simulink model "VCMGCM1962020b_v2"  (R2020b)
settings: Solver=FixedStepDiscrete  StartTime=0.0  StopTime=10.0  FixedStep=0.005  RelTol=1e-3  EnableMultiTasking=on
PreLoadFcn:
  | try, model_open; catch, disp('Error occurred while executing model pre-load callback: model_open.m'); disp('Please assure that the MATLAB working directory is set to the model directory before opening.'); end
InitFcn:
  | try, model_open; catch, end
undefined symbols (not defined in the file): Bridge, GCM, H, raptor_get_param_eval, raptor_get_safe_string, raptor_xcp_function
libraries: Blocks_lib x1165, Raptor_lib x665, simulink x62, VCM_lib x5
(part 11 of 23)

== system VCMGCM1962020b_v2/Fgnd/Sensors/CAN/Battery/DM01 ==
  note: The current .dbc, rev 6.0 has more messages than .dbc rev 4.0.
      | Have to figure out how these messages need to be routed.
  DiagEnbl : Inport
  Bus Creator : BusCreator  Inputs=2
  CANRxField5 : Blocks_lib/CANRxField  typ='uint8'  custom=off  custom_nam='---'  custom_units='---'
  CANRxMsgStatus : Blocks_lib/CANRxMsgStatus  samptime=samptime  custom=off  custom_nam='Name'  msgnam=DM01
  Ground : Ground
  Header : Blocks_lib/Header  width=Landscape  addtext=''
  raptor_can_rxmsg : Raptor_lib/CAN/raptor_can_rxmsg  canDefinition=struct('dbcFile', 'BMS dbc file_rev6.0.dbc','message', 'DM01','comment', '','signals', {{'Protect_Lamp','Amber_Warning_lamp','Red_Stop_Lamp','Malfunction_Indicator_Lamp','Flash_Protect_Lamp','Flash_Amber_Warning_Lamp','Flash_Red_Stop_Lamp','Flash_Malfunction_Indicator_Lamp','Suspect_Parameter_Number','Failure_Mode_Identifier','Occurence_Count','SPN_Conversion_Method'}},'enabled', [ 0 0 0 0 0 0 0 0 0 0 0 0;],'scaled', [ 1 1 1 1 1 1 1 1 1 1 1 1;],'canBus', 'bus','messageID', [ 419351283;],'idMask', [ 536870911;],'payloadMask', [],'payloadValue', [],'period', [ 0;],'mailbox', '''''','queueSize', [ 1;],'label', [ 1;],'ver', [ 2;],'showID', [ 0;],'showRaw', [ 0;],'fill', [ 0;],'editID', [ 0;],'signalOrder', [ 3;],'signalAscDes', [ 1;])  canBus=bus  mailbox=''  payloadMask=[]  payloadValue=[]  idMask=hex2dec('1FFFFFFF')  queueSize=1  showID=0  label=1  fill=0  id=419351283  showRaw=0  showAge=1  signalOrder=3  signalInfo={{struct('Name', 'Protect_Lamp','Startbit', [ 0;],'SignalSize', [ 4;],'ByteOrder', 'LittleEndian','ValueType', 'UNSIGNED','Class', 'uint8','Signed', [ 0;],'Factor', [ 1;],'Offset', [ 0;],'Min', [ 0;],'Max', [ 0;],'Units', '','Comment', '','StartBit', [ 0;]),struct('Name', 'Amber_Warning_lamp','Startbit', [ 0;],'SignalSize', [ 4;],'ByteOrder', 'LittleEndian','ValueType', 'UNSIGNED','Class', 'uint8','Signed', [ 0;],'Factor', [ 1;],'Offset', [ 0;],'Min', [ 0;],'Max', [ 0;],'Units', '','Comment', '','StartBit', [ 4;]),struct('Name', 'Red_Stop_Lamp','Startbit', [ 0;],'SignalSize', [ 4;],'ByteOrder', 'LittleEndian','ValueType', 'UNSIGNED','Class', 'uint8','Signed', [ 0;],'Factor', [ 1;],'Offset', [ 0;],'Min', [ 0;],'Max', [ 0;],'Units', '','Comment', '','StartBit', [ 8;]),struct('Name', 'Malfunction_Indicator_Lamp','Startbit', [ 0;],'SignalSize', [ 4;],'ByteOrder', 'LittleEndian','ValueType', 'UNSIGNED','Class', 'uint8','Signed', [ 0;],'Factor', [ 1;],'Offset', [ 0;],'Min', [ 0;],'Max', [ 0;],'Units', '','Comment', '','StartBit', [ 12;]),struct('Name', 'Flash_Protect_Lamp','Startbit', [ 0;],'SignalSize', [ 4;],'ByteOrder', 'LittleEndian','ValueType', 'UNSIGNED','Class', 'uint8','Signed', [ 0;],'Factor', [ 1;],'Offset', [ 0;],'Min', [ 0;],'Max', [ 0;],'Units', '','Comment', '','StartBit', [ 16;]),struct('Name', 'Flash_Amber_Warning_Lamp','Startbit', [ 0;],'SignalSize', [ 4;],'ByteOrder', 'LittleEndian','ValueType', 'UNSIGNED','Class', 'uint8','Signed', [ 0;],'Factor', [ 1;],'Offset', [ 0;],'Min', [ 0;],'Max', [ 0;],'Units', '','Comment', '','StartBit', [ 20;]),struct('Name', 'Flash_Red_Stop_Lamp','Startbit', [ 0;],'SignalSize', [ 4;],'ByteOrder', 'LittleEndian','ValueType', 'UNSIGNED','Class', 'uint8','Signed', [ 0;],'Factor', [ 1;],'Offset', [ 0;],'Min', [ 0;],'Max', [ 0;],'Units', '','Comment', '','StartBit', [ 24;]),struct('Name', 'Flash_Malfunction_Indicator_Lamp','Startbit', [ 0;],'SignalSize', [ 4;],'ByteOrder', 'LittleEndian','ValueType', 'UNSIGNED','Class', 'uint8','Signed', [ 0;],'Factor', [ 1;],'Offset', [ 0;],'Min', [ 0;],'Max', [ 0;],'Units', '','Comment', '','StartBit', [ 28;]),struct('Name', 'Suspect_Parameter_Number','Startbit', [ 0;],'SignalSize', [ 4;],'ByteOrder', 'LittleEndian','ValueType', 'UNSIGNED','Class', 'uint8','Signed', [ 0;],'Factor', [ 1;],'Offset', [ 0;],'Min', [ 0;],'Max', [ 0;],'Units', '','Comment', '','StartBit', [ 32;]),struct('Name', 'Failure_Mode_Identifier','Startbit', [ 0;],'SignalSize', [ 4;],'ByteOrder', 'LittleEndian','ValueType', 'UNSIGNED','Class', 'uint8','Signed', [ 0;],'Factor', [ 1;],'Offset', [ 0;],'Min', [ 0;],'Max', [ 0;],'Units', '','Comment', '','StartBit', [ 36;]),struct('Name', 'Occurence_Count','Startbit', [ 0;],'SignalSize', [ 4;],'ByteOrder', 'LittleEndian','ValueType', 'UNSIGNED','Class', 'uint8','Signed', [ 0;],'Factor', [ 1;],'Offset', [ 0;],'Min', [ 0;],'Max', [ 0;],'Units', '','Comment', '','StartBit', [ 40;]),struct('Name', 'SPN_Conversion_Method','Startbit', [ 0;],'SignalSize', [ 4;],'ByteOrder', 'LittleEndian','ValueType', 'UNSIGNED','Class', 'uint8','Signed', [ 0;],'Factor', [ 1;],'Offset', [ 0;],'Min', [ 0;],'Max', [ 0;],'Units', '','Comment', '','StartBit', [ 44;])}}
      settings: SourceProductName=Raptor
  Data : Outport  VectorParamsAs1DForOutWhenUnconnected=off
  wires:
  Bus Creator/1 -> Data/1  "MsgName"
  CANRxMsgStatus/1 -> Bus Creator/1
  DiagEnbl/1 -> CANRxMsgStatus/1
  raptor_can_rxmsg/1 -> CANRxMsgStatus/2  "Age"
  CANRxField5/1 -> Bus Creator/2
  Ground/1 -> CANRxField5/1  "Fault"

== system VCMGCM1962020b_v2/Fgnd/Sensors/CAN/Battery/HVES1_Data1 ==
  DiagEnbl : Inport
  Bus Creator : BusCreator  Inputs=5
  CANRxField{,1..3} (4 alike) : Blocks_lib/CANRxField  typ='double'  custom=off  custom_nam='---'  custom_units='---'
  CANRxMsgStatus : Blocks_lib/CANRxMsgStatus  samptime=samptime  custom=off  custom_nam='Name'  msgnam=HVES1_Data1
  Header : Blocks_lib/Header  width=Landscape  addtext=''
  raptor_can_rxmsg : Raptor_lib/CAN/raptor_can_rxmsg  canDefinition=struct('dbcFile', 'BMS dbc file_rev4.0.dbc','message', 'HVES1_Data1','comment', '20ms','signals', {{'Batt_Disch_Pow','Batt_Char_Pow','Batt_Voltage','Batt_Current'}},'enabled', [ 1 1 1 1;],'scaled', [ 1 1 1 1;],'canBus', 'bus','messageID', [ 217092339;],'idMask', [ 536870911;],'payloadMask', [],'payloadValue', [],'period', [ 0;],'mailbox', '''''','queueSize', [ 1;],'label', [ 1;],'ver', [ 2;],'showID', [ 0;],'showRaw', [ 0;],'showRawMsg', [ 0;],'showAge', [ 1;],'fill', [ 0;],'editID', [ 0;],'signalOrder', [ 3;],'signalAscDes', [ 1;])  canBus=bus  mailbox=''  payloadMask=[]  payloadValue=[]  idMask=hex2dec('1FFFFFFF')  queueSize=1  showID=0  label=1  fill=0  id=217092339  showRaw=0  showAge=1  signalOrder=3  signalInfo={{struct('Name', 'Batt_Disch_Pow','Startbit', [ 0;],'SignalSize', [ 16;],'ByteOrder', 'LittleEndian','ValueType', 'UNSIGNED','Class', 'uint16','Signed', [ 0;],'Factor', [ 0.05;],'Offset', [ 0;],'Min', [ 0;],'Max', [ 3212.75;],'Units', 'kW','Comment', '','StartBit', [ 0;]),struct('Name', 'Batt_Char_Pow','Startbit', [ 0;],'SignalSize', [ 16;],'ByteOrder', 'LittleEndian','ValueType', 'UNSIGNED','Class', 'uint16','Signed', [ 0;],'Factor', [ 0.05;],'Offset', [ 0;],'Min', [ 0;],'Max', [ 3212.75;],'Units', 'kW','Comment', '','StartBit', [ 16;]),struct('Name', 'Batt_Voltage','Startbit', [ 0;],'SignalSize', [ 16;],'ByteOrder', 'LittleEndian','ValueType', 'UNSIGNED','Class', 'uint16','Signed', [ 0;],'Factor', [ 0.05;],'Offset', [ 0;],'Min', [ 0;],'Max', [ 3212.75;],'Units', 'V','Comment', '','StartBit', [ 32;]),struct('Name', 'Batt_Current','Startbit', [ 0;],'SignalSize', [ 16;],'ByteOrder', 'LittleEndian','ValueType', 'UNSIGNED','Class', 'uint16','Signed', [ 0;],'Factor', [ 0.05;],'Offset', [ -1600;],'Min', [ -1600;],'Max', [ 1612.75;],'Units', 'A','Comment', '','StartBit', [ 48;])}}
      settings: SourceProductName=Raptor
  Data : Outport  VectorParamsAs1DForOutWhenUnconnected=off
  wires:
  Bus Creator/1 -> Data/1  "MsgName"
  raptor_can_rxmsg/2 -> CANRxField/1  "Batt_Disch_Pow"
  CANRxMsgStatus/1 -> Bus Creator/1
  CANRxField/1 -> Bus Creator/2
  DiagEnbl/1 -> CANRxMsgStatus/1
  raptor_can_rxmsg/1 -> CANRxMsgStatus/2  "Age"
  raptor_can_rxmsg/5 -> CANRxField3/1  "Batt_Current"
  raptor_can_rxmsg/3 -> CANRxField1/1  "Batt_Char_Pow"
  raptor_can_rxmsg/4 -> CANRxField2/1  "Batt_Voltage"
  CANRxField1/1 -> Bus Creator/3
  CANRxField2/1 -> Bus Creator/4
  CANRxField3/1 -> Bus Creator/5

== system VCMGCM1962020b_v2/Fgnd/Sensors/CAN/Battery/HVES1_Data10 ==
  DiagEnbl : Inport
  Bus Creator : BusCreator  Inputs=2
  CANRxField : Blocks_lib/CANRxField  typ='double'  custom=off  custom_nam='---'  custom_units='---'
  CANRxMsgStatus : Blocks_lib/CANRxMsgStatus  samptime=samptime  custom=off  custom_nam='Name'  msgnam=HVES1_Data10
  Header : Blocks_lib/Header  width=Landscape  addtext=''
  raptor_can_rxmsg : Raptor_lib/CAN/raptor_can_rxmsg  canDefinition=struct('dbcFile', 'BMS dbc file_rev4.0.dbc','message', 'HVES1_Data10','comment', '100ms','signals', {{'PSV_ISO_Measurement'}},'enabled', [ 1;],'scaled', [ 1;],'canBus', 'bus','messageID', [ 217124083;],'idMask', [ 536870911;],'payloadMask', [],'payloadValue', [],'period', [ 0;],'mailbox', '''''','queueSize', [ 1;],'label', [ 1;],'ver', [ 2;],'showID', [ 0;],'showRaw', [ 0;],'showRawMsg', [ 0;],'showAge', [ 1;],'fill', [ 0;],'editID', [ 0;],'signalOrder', [ 3;],'signalAscDes', [ 1;])  canBus=bus  mailbox=''  payloadMask=[]  payloadValue=[]  idMask=hex2dec('1FFFFFFF')  queueSize=1  showID=0  label=1  fill=0  id=217124083  showRaw=0  showAge=1  signalOrder=3  signalInfo={{struct('Name', 'PSV_ISO_Measurement','Startbit', [ 0;],'SignalSize', [ 16;],'ByteOrder', 'LittleEndian','ValueType', 'UNSIGNED','Class', 'uint16','Signed', [ 0;],'Factor', [ 0.1;],'Offset', [ 0;],'Min', [ 0;],'Max', [ 6425.5;],'Units', 'ohm/volt','Comment', '','StartBit', [ 48;])}}
      settings: SourceProductName=Raptor
  Data : Outport  VectorParamsAs1DForOutWhenUnconnected=off
  wires:
  Bus Creator/1 -> Data/1  "MsgName"
  raptor_can_rxmsg/2 -> CANRxField/1  "PSV_ISO_Measurement"
  CANRxMsgStatus/1 -> Bus Creator/1
  CANRxField/1 -> Bus Creator/2
  DiagEnbl/1 -> CANRxMsgStatus/1
  raptor_can_rxmsg/1 -> CANRxMsgStatus/2  "Age"

== system VCMGCM1962020b_v2/Fgnd/Sensors/CAN/Battery/HVES1_Data2 ==
  DiagEnbl : Inport
  Bus Creator : BusCreator  Inputs=4
  CANRxField : Blocks_lib/CANRxField  typ='double'  custom=off  custom_nam='---'  custom_units='---'
  CANRxField1 : Blocks_lib/CANRxField  typ='double'  custom=off  custom_nam='---'  custom_units='---'
  CANRxField2 : Blocks_lib/CANRxField  typ='double'  custom=off  custom_nam='---'  custom_units='---'
  CANRxMsgStatus : Blocks_lib/CANRxMsgStatus  samptime=samptime  custom=off  custom_nam='Name'  msgnam=HVES1_Data2
  Header : Blocks_lib/Header  width=Landscape  addtext=''
  raptor_can_rxmsg : Raptor_lib/CAN/raptor_can_rxmsg  canDefinition=struct('dbcFile', 'BMS dbc file_rev4.0.dbc','message', 'HVES1_Data2','comment', '20ms','signals', {{'Batt_SOC','Batt_Cell_Volt_High','Batt_Cell_Volt_Low'}},'enabled', [ 1 1 1;],'scaled', [ 1 1 1;],'canBus', 'bus','messageID', [ 217092595;],'idMask', [ 536870911;],'payloadMask', [],'payloadValue', [],'period', [ 0;],'mailbox', '''''','queueSize', [ 1;],'label', [ 1;],'ver', [ 2;],'showID', [ 0;],'showRaw', [ 0;],'showRawMsg', [ 0;],'showAge', [ 1;],'fill', [ 0;],'editID', [ 0;],'signalOrder', [ 3;],'signalAscDes', [ 1;])  canBus=bus  mailbox=''  payloadMask=[]  payloadValue=[]  idMask=hex2dec('1FFFFFFF')  queueSize=1  showID=0  label=1  fill=0  id=217092595  showRaw=0  showAge=1  signalOrder=3  signalInfo={{struct('Name', 'Batt_SOC','Startbit', [ 0;],'SignalSize', [ 16;],'ByteOrder', 'LittleEndian','ValueType', 'UNSIGNED','Class', 'uint16','Signed', [ 0;],'Factor', [ 0.0015625;],'Offset', [ 0;],'Min', [ 0;],'Max', [ 100.3984;],'Units', '%','Comment', '','StartBit', [ 0;]),struct('Name', 'Batt_Cell_Volt_High','Startbit', [ 0;],'SignalSize', [ 16;],'ByteOrder', 'LittleEndian','ValueType', 'UNSIGNED','Class', 'uint16','Signed', [ 0;],'Factor', [ 0.001;],'Offset', [ 0;],'Min', [ 0;],'Max', [ 64.225;],'Units', 'V','Comment', '','StartBit', [ 16;]),struct('Name', 'Batt_Cell_Volt_Low','Startbit', [ 0;],'SignalSize', [ 16;],'ByteOrder', 'LittleEndian','ValueType', 'UNSIGNED','Class', 'uint16','Signed', [ 0;],'Factor', [ 0.001;],'Offset', [ 0;],'Min', [ 0;],'Max', [ 64.225;],'Units', 'V','Comment', '','StartBit', [ 32;])}}
      settings: SourceProductName=Raptor
  Data : Outport  VectorParamsAs1DForOutWhenUnconnected=off
  wires:
  Bus Creator/1 -> Data/1  "MsgName"
  raptor_can_rxmsg/2 -> CANRxField/1  "Batt_SOC"
  CANRxMsgStatus/1 -> Bus Creator/1
  CANRxField/1 -> Bus Creator/2
  DiagEnbl/1 -> CANRxMsgStatus/1
  raptor_can_rxmsg/1 -> CANRxMsgStatus/2  "Age"
  raptor_can_rxmsg/3 -> CANRxField1/1  "Batt_Cell_Volt_High"
  raptor_can_rxmsg/4 -> CANRxField2/1  "Batt_Cell_Volt_Low"
  CANRxField1/1 -> Bus Creator/3
  CANRxField2/1 -> Bus Creator/4

== system VCMGCM1962020b_v2/Fgnd/Sensors/CAN/Battery/HVES1_Data3 ==
  DiagEnbl : Inport
  Bus Creator : BusCreator  Inputs=4
  CANRxField : Blocks_lib/CANRxField  typ='double'  custom=off  custom_nam='---'  custom_units='---'
  CANRxField1 : Blocks_lib/CANRxField  typ='double'  custom=off  custom_nam='---'  custom_units='---'
  CANRxField2 : Blocks_lib/CANRxField  typ='double'  custom=off  custom_nam='---'  custom_units='---'
  CANRxMsgStatus : Blocks_lib/CANRxMsgStatus  samptime=samptime  custom=off  custom_nam='Name'  msgnam=HVES1_Data3
  Header : Blocks_lib/Header  width=Landscape  addtext=''
  raptor_can_rxmsg : Raptor_lib/CAN/raptor_can_rxmsg  canDefinition=struct('dbcFile', 'BMS dbc file_rev4.0.dbc','message', 'HVES1_Data3','comment', '20ms','signals', {{'Batt_Max_Cell_Temp','Batt_Min_Cell_Temp','Batt_Ave_Cell_Temp'}},'enabled', [ 1 1 1;],'scaled', [ 1 1 1;],'canBus', 'bus','messageID', [ 217092851;],'idMask', [ 536870911;],'payloadMask', [],'payloadValue', [],'period', [ 0;],'mailbox', '''''','queueSize', [ 1;],'label', [ 1;],'ver', [ 2;],'showID', [ 0;],'showRaw', [ 0;],'showRawMsg', [ 0;],'showAge', [ 1;],'fill', [ 0;],'editID', [ 0;],'signalOrder', [ 3;],'signalAscDes', [ 1;])  canBus=bus  mailbox=''  payloadMask=[]  payloadValue=[]  idMask=hex2dec('1FFFFFFF')  queueSize=1  showID=0  label=1  fill=0  id=217092851  showRaw=0  showAge=1  signalOrder=3  signalInfo={{struct('Name', 'Batt_Max_Cell_Temp','Startbit', [ 0;],'SignalSize', [ 16;],'ByteOrder', 'LittleEndian','ValueType', 'UNSIGNED','Class', 'uint16','Signed', [ 0;],'Factor', [ 0.03125;],'Offset', [ -273;],'Min', [ -273;],'Max', [ 1734.9687;],'Units', 'C','Comment', '','StartBit', [ 0;]),struct('Name', 'Batt_Min_Cell_Temp','Startbit', [ 0;],'SignalSize', [ 16;],'ByteOrder', 'LittleEndian','ValueType', 'UNSIGNED','Class', 'uint16','Signed', [ 0;],'Factor', [ 0.03125;],'Offset', [ -273;],'Min', [ -273;],'Max', [ 1734.9688;],'Units', 'C','Comment', '','StartBit', [ 16;]),struct('Name', 'Batt_Ave_Cell_Temp','Startbit', [ 0;],'SignalSize', [ 16;],'ByteOrder', 'LittleEndian','ValueType', 'UNSIGNED','Class', 'uint16','Signed', [ 0;],'Factor', [ 0.03125;],'Offset', [ -273;],'Min', [ -273;],'Max', [ 1734.9688;],'Units', 'C','Comment', '','StartBit', [ 32;])}}
      settings: SourceProductName=Raptor
  Data : Outport  VectorParamsAs1DForOutWhenUnconnected=off
  wires:
  Bus Creator/1 -> Data/1  "MsgName"
  raptor_can_rxmsg/2 -> CANRxField/1  "Batt_Max_Cell_Temp"
  CANRxMsgStatus/1 -> Bus Creator/1
  CANRxField/1 -> Bus Creator/2
  DiagEnbl/1 -> CANRxMsgStatus/1
  raptor_can_rxmsg/1 -> CANRxMsgStatus/2  "Age"
  raptor_can_rxmsg/3 -> CANRxField1/1  "Batt_Min_Cell_Temp"
  raptor_can_rxmsg/4 -> CANRxField2/1  "Batt_Ave_Cell_Temp"
  CANRxField1/1 -> Bus Creator/3
  CANRxField2/1 -> Bus Creator/4

== system VCMGCM1962020b_v2/Fgnd/Sensors/CAN/Battery/HVES1_Data4 ==
  DiagEnbl : Inport
  Bus Creator : BusCreator  Inputs=3
  CANRxField : Blocks_lib/CANRxField  typ='double'  custom=off  custom_nam='---'  custom_units='---'
  CANRxField1 : Blocks_lib/CANRxField  typ='double'  custom=off  custom_nam='---'  custom_units='---'
  CANRxMsgStatus : Blocks_lib/CANRxMsgStatus  samptime=samptime  custom=off  custom_nam='Name'  msgnam=HVES1_Data4
  Header : Blocks_lib/Header  width=Landscape  addtext=''
  raptor_can_rxmsg : Raptor_lib/CAN/raptor_can_rxmsg  canDefinition=struct('dbcFile', 'BMS dbc file_rev4.0.dbc','message', 'HVES1_Data4','comment', '100ms','signals', {{'Batt_Disch_cap','Batt_Charge_cap'}},'enabled', [ 1 1;],'scaled', [ 1 1;],'canBus', 'bus','messageID', [ 217093107;],'idMask', [ 536870911;],'payloadMask', [],'payloadValue', [],'period', [ 0;],'mailbox', '''''','queueSize', [ 1;],'label', [ 1;],'ver', [ 2;],'showID', [ 0;],'showRaw', [ 0;],'showRawMsg', [ 0;],'showAge', [ 1;],'fill', [ 0;],'editID', [ 0;],'signalOrder', [ 3;],'signalAscDes', [ 1;])  canBus=bus  mailbox=''  payloadMask=[]  payloadValue=[]  idMask=hex2dec('1FFFFFFF')  queueSize=1  showID=0  label=1  fill=0  id=217093107  showRaw=0  showAge=1  signalOrder=3  signalInfo={{struct('Name', 'Batt_Disch_cap','Startbit', [ 0;],'SignalSize', [ 16;],'ByteOrder', 'LittleEndian','ValueType', 'UNSIGNED','Class', 'uint16','Signed', [ 0;],'Factor', [ 0.01;],'Offset', [ 0;],'Min', [ 0;],'Max', [ 642.55;],'Units', 'Ah','Comment', '','StartBit', [ 0;]),struct('Name', 'Batt_Charge_cap','Startbit', [ 0;],'SignalSize', [ 16;],'ByteOrder', 'LittleEndian','ValueType', 'UNSIGNED','Class', 'uint16','Signed', [ 0;],'Factor', [ 0.01;],'Offset', [ 0;],'Min', [ 0;],'Max', [ 642.55;],'Units', 'Ah','Comment', '','StartBit', [ 16;])}}
      settings: SourceProductName=Raptor
  Data : Outport  VectorParamsAs1DForOutWhenUnconnected=off
  wires:
  Bus Creator/1 -> Data/1  "MsgName"
  raptor_can_rxmsg/2 -> CANRxField/1  "Batt_Disch_cap"
  CANRxMsgStatus/1 -> Bus Creator/1
  CANRxField/1 -> Bus Creator/2
  DiagEnbl/1 -> CANRxMsgStatus/1
  raptor_can_rxmsg/1 -> CANRxMsgStatus/2  "Age"
  raptor_can_rxmsg/3 -> CANRxField1/1  "Batt_Charge_cap"
  CANRxField1/1 -> Bus Creator/3

== system VCMGCM1962020b_v2/Fgnd/Sensors/CAN/Battery/HVES1_Data5 ==
  DiagEnbl : Inport
  Bus Creator : BusCreator  Inputs=3
  CANRxField : Blocks_lib/CANRxField  typ='double'  custom=off  custom_nam='---'  custom_units='---'
  CANRxField1 : Blocks_lib/CANRxField  typ='double'  custom=off  custom_nam='---'  custom_units='---'
  CANRxMsgStatus : Blocks_lib/CANRxMsgStatus  samptime=samptime  custom=off  custom_nam='Name'  msgnam=HVES1_Data5
  Header : Blocks_lib/Header  width=Landscape  addtext=''
  raptor_can_rxmsg : Raptor_lib/CAN/raptor_can_rxmsg  canDefinition=struct('dbcFile', 'BMS dbc file_rev4.0.dbc','message', 'HVES1_Data5','comment', '20ms','signals', {{'Batt_Disch_Curr_Lim','Batt_Charge_Curr_Lim'}},'enabled', [ 1 1;],'scaled', [ 1 1;],'canBus', 'bus','messageID', [ 217093363;],'idMask', [ 536870911;],'payloadMask', [],'payloadValue', [],'period', [ 0;],'mailbox', '''''','queueSize', [ 1;],'label', [ 1;],'ver', [ 2;],'showID', [ 0;],'showRaw', [ 0;],'showRawMsg', [ 0;],'showAge', [ 1;],'fill', [ 0;],'editID', [ 0;],'signalOrder', [ 3;],'signalAscDes', [ 1;])  canBus=bus  mailbox=''  payloadMask=[]  payloadValue=[]  idMask=hex2dec('1FFFFFFF')  queueSize=1  showID=0  label=1  fill=0  id=217093363  showRaw=0  showAge=1  signalOrder=3  signalInfo={{struct('Name', 'Batt_Disch_Curr_Lim','Startbit', [ 0;],'SignalSize', [ 16;],'ByteOrder', 'LittleEndian','ValueType', 'UNSIGNED','Class', 'uint16','Signed', [ 0;],'Factor', [ 0.05;],'Offset', [ -1600;],'Min', [ -1600;],'Max', [ 1612.75;],'Units', 'A','Comment', '','StartBit', [ 0;]),struct('Name', 'Batt_Charge_Curr_Lim','Startbit', [ 0;],'SignalSize', [ 16;],'ByteOrder', 'LittleEndian','ValueType', 'UNSIGNED','Class', 'uint16','Signed', [ 0;],'Factor', [ 0.05;],'Offset', [ -1600;],'Min', [ -1600;],'Max', [ 1612.75;],'Units', 'A','Comment', '','StartBit', [ 16;])}}
      settings: SourceProductName=Raptor
  Data : Outport  VectorParamsAs1DForOutWhenUnconnected=off
  wires:
  Bus Creator/1 -> Data/1  "MsgName"
  raptor_can_rxmsg/2 -> CANRxField/1  "Batt_Disch_Curr_Lim"
  CANRxMsgStatus/1 -> Bus Creator/1
  CANRxField/1 -> Bus Creator/2
  DiagEnbl/1 -> CANRxMsgStatus/1
  raptor_can_rxmsg/1 -> CANRxMsgStatus/2  "Age"
  raptor_can_rxmsg/3 -> CANRxField1/1  "Batt_Charge_Curr_Lim"
  CANRxField1/1 -> Bus Creator/3

== system VCMGCM1962020b_v2/Fgnd/Sensors/CAN/Battery/HVES1_Data6 ==
  DiagEnbl : Inport
  Bus Creator : BusCreator  Inputs=4
  CANRxField : Blocks_lib/CANRxField  typ='double'  custom=off  custom_nam='---'  custom_units='---'
  CANRxField1 : Blocks_lib/CANRxField  typ='double'  custom=off  custom_nam='---'  custom_units='---'
  CANRxField2 : Blocks_lib/CANRxField  typ='double'  custom=off  custom_nam='---'  custom_units='---'
  CANRxMsgStatus : Blocks_lib/CANRxMsgStatus  samptime=samptime  custom=off  custom_nam='Name'  msgnam=HVES1_Data6
  Header : Blocks_lib/Header  width=Landscape  addtext=''
  raptor_can_rxmsg : Raptor_lib/CAN/raptor_can_rxmsg  canDefinition=struct('dbcFile', 'BMS dbc file_rev4.0.dbc','message', 'HVES1_Data6','comment', '100ms','signals', {{'Batt_Bus_Vol','Batt_inlet_cool_temp','Batt_outlet_cool_temp'}},'enabled', [ 1 1 1;],'scaled', [ 1 1 1;],'canBus', 'bus','messageID', [ 217093619;],'idMask', [ 536870911;],'payloadMask', [],'payloadValue', [],'period', [ 0;],'mailbox', '''''','queueSize', [ 1;],'label', [ 1;],'ver', [ 2;],'showID', [ 0;],'showRaw', [ 0;],'showRawMsg', [ 0;],'showAge', [ 1;],'fill', [ 0;],'editID', [ 0;],'signalOrder', [ 3;],'signalAscDes', [ 1;])  canBus=bus  mailbox=''  payloadMask=[]  payloadValue=[]  idMask=hex2dec('1FFFFFFF')  queueSize=1  showID=0  label=1  fill=0  id=217093619  showRaw=0  showAge=1  signalOrder=3  signalInfo={{struct('Name', 'Batt_Bus_Vol','Startbit', [ 0;],'SignalSize', [ 16;],'ByteOrder', 'LittleEndian','ValueType', 'UNSIGNED','Class', 'uint16','Signed', [ 0;],'Factor', [ 0.05;],'Offset', [ 0;],'Min', [ 0;],'Max', [ 3212.75;],'Units', 'V','Comment', '','StartBit', [ 0;]),struct('Name', 'Batt_inlet_cool_temp','Startbit', [ 0;],'SignalSize', [ 8;],'ByteOrder', 'LittleEndian','ValueType', 'UNSIGNED','Class', 'uint8','Signed', [ 0;],'Factor', [ 1;],'Offset', [ -40;],'Min', [ -40;],'Max', [ 210;],'Units', 'C','Comment', '','StartBit', [ 32;]),struct('Name', 'Batt_outlet_cool_temp','Startbit', [ 0;],'SignalSize', [ 8;],'ByteOrder', 'LittleEndian','ValueType', 'UNSIGNED','Class', 'uint8','Signed', [ 0;],'Factor', [ 1;],'Offset', [ -40;],'Min', [ -40;],'Max', [ 210;],'Units', 'C','Comment', '','StartBit', [ 40;])}}
      settings: SourceProductName=Raptor
  Data : Outport  VectorParamsAs1DForOutWhenUnconnected=off
  wires:
  Bus Creator/1 -> Data/1  "MsgName"
  raptor_can_rxmsg/2 -> CANRxField/1  "Batt_Bus_Vol"
  CANRxMsgStatus/1 -> Bus Creator/1
  CANRxField/1 -> Bus Creator/2
  DiagEnbl/1 -> CANRxMsgStatus/1
  raptor_can_rxmsg/1 -> CANRxMsgStatus/2  "Age"
  raptor_can_rxmsg/3 -> CANRxField1/1  "Batt_inlet_cool_temp"
  CANRxField1/1 -> Bus Creator/3
  raptor_can_rxmsg/4 -> CANRxField2/1  "Batt_outlet_cool_temp"
  CANRxField2/1 -> Bus Creator/4

== system VCMGCM1962020b_v2/Fgnd/Sensors/CAN/Battery/HVES1_Data7 ==
  DiagEnbl : Inport
  Bus Creator : BusCreator  Inputs=4
  CANRxField : Blocks_lib/CANRxField  typ='double'  custom=off  custom_nam='---'  custom_units='---'
  CANRxField1 : Blocks_lib/CANRxField  typ='double'  custom=off  custom_nam='---'  custom_units='---'
  CANRxField2 : Blocks_lib/CANRxField  typ='double'  custom=off  custom_nam='---'  custom_units='---'
  CANRxMsgStatus : Blocks_lib/CANRxMsgStatus  samptime=samptime  custom=off  custom_nam='Name'  msgnam=HVES1_Data7
  Header : Blocks_lib/Header  width=Landscape  addtext=''
  raptor_can_rxmsg : Raptor_lib/CAN/raptor_can_rxmsg  canDefinition=struct('dbcFile', 'BMS dbc file_rev4.0.dbc','message', 'HVES1_Data7','comment', '100ms','signals', {{'Batt_Dchg_Ene','Batt_Chg_Ene','Batt_Max_Vol'}},'enabled', [ 1 1 1;],'scaled', [ 1 1 1;],'canBus', 'bus','messageID', [ 217096435;],'idMask', [ 536870911;],'payloadMask', [],'payloadValue', [],'period', [ 0;],'mailbox', '''''','queueSize', [ 1;],'label', [ 1;],'ver', [ 2;],'showID', [ 0;],'showRaw', [ 0;],'showRawMsg', [ 0;],'showAge', [ 1;],'fill', [ 0;],'editID', [ 0;],'signalOrder', [ 3;],'signalAscDes', [ 1;])  canBus=bus  mailbox=''  payloadMask=[]  payloadValue=[]  idMask=hex2dec('1FFFFFFF')  queueSize=1  showID=0  label=1  fill=0  id=217096435  showRaw=0  showAge=1  signalOrder=3  signalInfo={{struct('Name', 'Batt_Dchg_Ene','Startbit', [ 0;],'SignalSize', [ 24;],'ByteOrder', 'LittleEndian','ValueType', 'UNSIGNED','Class', 'uint32','Signed', [ 0;],'Factor', [ 0.001;],'Offset', [ 0;],'Min', [ 0;],'Max', [ 16449.535;],'Units', 'kWh','Comment', '','StartBit', [ 0;]),struct('Name', 'Batt_Chg_Ene','Startbit', [ 0;],'SignalSize', [ 24;],'ByteOrder', 'LittleEndian','ValueType', 'UNSIGNED','Class', 'uint32','Signed', [ 0;],'Factor', [ 0.001;],'Offset', [ 0;],'Min', [ 0;],'Max', [ 16499.535;],'Units', 'kWh','Comment', '','StartBit', [ 24;]),struct('Name', 'Batt_Max_Vol','Startbit', [ 0;],'SignalSize', [ 16;],'ByteOrder', 'LittleEndian','ValueType', 'UNSIGNED','Class', 'uint16','Signed', [ 0;],'Factor', [ 0.05;],'Offset', [ 0;],'Min', [ 0;],'Max', [ 3212.75;],'Units', 'V','Comment', '','StartBit', [ 48;])}}
      settings: SourceProductName=Raptor
  Data : Outport  VectorParamsAs1DForOutWhenUnconnected=off
  wires:
  Bus Creator/1 -> Data/1  "MsgName"
  raptor_can_rxmsg/2 -> CANRxField/1  "Batt_Dchg_Ene"
  CANRxMsgStatus/1 -> Bus Creator/1
  CANRxField/1 -> Bus Creator/2
  DiagEnbl/1 -> CANRxMsgStatus/1
  raptor_can_rxmsg/1 -> CANRxMsgStatus/2  "Age"
  raptor_can_rxmsg/3 -> CANRxField1/1  "Batt_Chg_Ene"
  CANRxField1/1 -> Bus Creator/3
  raptor_can_rxmsg/4 -> CANRxField2/1  "Batt_Max_Vol"
  CANRxField2/1 -> Bus Creator/4

== system VCMGCM1962020b_v2/Fgnd/Sensors/CAN/Battery/HVES1_Data8 ==
  DiagEnbl : Inport
  Bus Creator : BusCreator  Inputs=2
  CANRxField : Blocks_lib/CANRxField  typ='double'  custom=off  custom_nam='---'  custom_units='---'
  CANRxMsgStatus : Blocks_lib/CANRxMsgStatus  samptime=samptime  custom=off  custom_nam='Name'  msgnam=HVES1_Data8
  Header : Blocks_lib/Header  width=Landscape  addtext=''
  raptor_can_rxmsg : Raptor_lib/CAN/raptor_can_rxmsg  canDefinition=struct('dbcFile', 'BMS dbc file_rev4.0.dbc','message', 'HVES1_Data8','comment', '100ms','signals', {{'Batt_Cell_Vol'}},'enabled', [ 1;],'scaled', [ 1;],'canBus', 'bus','messageID', [ 217123571;],'idMask', [ 536870911;],'payloadMask', [],'payloadValue', [],'period', [ 0;],'mailbox', '''''','queueSize', [ 1;],'label', [ 1;],'ver', [ 2;],'showID', [ 0;],'showRaw', [ 0;],'showRawMsg', [ 0;],'showAge', [ 1;],'fill', [ 0;],'editID', [ 0;],'signalOrder', [ 3;],'signalAscDes', [ 1;])  canBus=bus  mailbox=''  payloadMask=[]  payloadValue=[]  idMask=hex2dec('1FFFFFFF')  queueSize=1  showID=0  label=1  fill=0  id=217123571  showRaw=0  showAge=1  signalOrder=3  signalInfo={{struct('Name', 'Batt_Cell_Vol','Startbit', [ 0;],'SignalSize', [ 16;],'ByteOrder', 'LittleEndian','ValueType', 'UNSIGNED','Class', 'uint16','Signed', [ 0;],'Factor', [ 0.001;],'Offset', [ 0;],'Min', [ 0;],'Max', [ 64.255;],'Units', 'V','Comment', '','StartBit', [ 32;])}}
      settings: SourceProductName=Raptor
  Data : Outport  VectorParamsAs1DForOutWhenUnconnected=off
  wires:
  Bus Creator/1 -> Data/1  "MsgName"
  raptor_can_rxmsg/2 -> CANRxField/1  "Batt_Cell_Vol"
  CANRxMsgStatus/1 -> Bus Creator/1
  CANRxField/1 -> Bus Creator/2
  DiagEnbl/1 -> CANRxMsgStatus/1
  raptor_can_rxmsg/1 -> CANRxMsgStatus/2  "Age"

== system VCMGCM1962020b_v2/Fgnd/Sensors/CAN/Battery/HVES1_HIST ==
  DiagEnbl : Inport
  Bus Creator : BusCreator  Inputs=4
  CANRxField : Blocks_lib/CANRxField  typ='double'  custom=off  custom_nam='---'  custom_units='---'
  CANRxField1 : Blocks_lib/CANRxField  typ='double'  custom=off  custom_nam='---'  custom_units='---'
  CANRxField2 : Blocks_lib/CANRxField  typ='double'  custom=off  custom_nam='---'  custom_units='---'
  CANRxMsgStatus : Blocks_lib/CANRxMsgStatus  samptime=samptime  custom=off  custom_nam='Name'  msgnam=HVES1_HIST
  Header : Blocks_lib/Header  width=Landscape  addtext=''
  raptor_can_rxmsg : Raptor_lib/CAN/raptor_can_rxmsg  canDefinition=struct('dbcFile', 'BMS dbc file_rev4.0.dbc','message', 'HVES1_HIST','comment', '100ms','signals', {{'Batt_SOH','Contactor_Open_UndrLoad','Batt_Total_Energy'}},'enabled', [ 1 1 1;],'scaled', [ 1 1 1;],'canBus', 'bus','messageID', [ 486301427;],'idMask', [ 536870911;],'payloadMask', [],'payloadValue', [],'period', [ 0;],'mailbox', '''''','queueSize', [ 1;],'label', [ 1;],'ver', [ 2;],'showID', [ 0;],'showRaw', [ 0;],'showRawMsg', [ 0;],'showAge', [ 1;],'fill', [ 0;],'editID', [ 0;],'signalOrder', [ 3;],'signalAscDes', [ 1;])  canBus=bus  mailbox=''  payloadMask=[]  payloadValue=[]  idMask=hex2dec('1FFFFFFF')  queueSize=1  showID=0  label=1  fill=0  id=486301427  showRaw=0  showAge=1  signalOrder=3  signalInfo={{struct('Name', 'Batt_SOH','Startbit', [ 0;],'SignalSize', [ 8;],'ByteOrder', 'LittleEndian','ValueType', 'UNSIGNED','Class', 'uint8','Signed', [ 0;],'Factor', [ 0.4;],'Offset', [ 0;],'Min', [ 0;],'Max', [ 100;],'Units', '%','Comment', '','StartBit', [ 0;]),struct('Name', 'Contactor_Open_UndrLoad','Startbit', [ 0;],'SignalSize', [ 16;],'ByteOrder', 'LittleEndian','ValueType', 'UNSIGNED','Class', 'uint16','Signed', [ 0;],'Factor', [ 1;],'Offset', [ 0;],'Min', [ 0;],'Max', [ 64255;],'Units', 'count','Comment', '','StartBit', [ 8;]),struct('Name', 'Batt_Total_Energy','Startbit', [ 0;],'SignalSize', [ 32;],'ByteOrder', 'LittleEndian','ValueType', 'UNSIGNED','Class', 'uint32','Signed', [ 0;],'Factor', [ 100;],'Offset', [ 0;],'Min', [ 0;],'Max', [ 421108121500;],'Units', 'Wh','Comment', '','StartBit', [ 24;])}}
      settings: SourceProductName=Raptor
  Data : Outport  VectorParamsAs1DForOutWhenUnconnected=off
  wires:
  Bus Creator/1 -> Data/1  "MsgName"
  raptor_can_rxmsg/2 -> CANRxField/1  "Batt_SOH"
  CANRxMsgStatus/1 -> Bus Creator/1
  CANRxField/1 -> Bus Creator/2
  DiagEnbl/1 -> CANRxMsgStatus/1
  raptor_can_rxmsg/1 -> CANRxMsgStatus/2  "Age"
  raptor_can_rxmsg/3 -> CANRxField1/1  "Contactor_Open_UndrLoad"
  raptor_can_rxmsg/4 -> CANRxField2/1  "Batt_Total_Energy"
  CANRxField1/1 -> Bus Creator/3
  CANRxField2/1 -> Bus Creator/4

== system VCMGCM1962020b_v2/Fgnd/Sensors/CAN/Battery/HVES1_Status1 ==
  DiagEnbl : Inport
  Bus Creator : BusCreator  Inputs=6
  CANRxField{,1..4} (5 alike) : Blocks_lib/CANRxField  typ='uint8'  custom=off  custom_nam='---'  custom_units='---'
  CANRxMsgStatus : Blocks_lib/CANRxMsgStatus  samptime=samptime  custom=off  custom_nam='Name'  msgnam=HVES1_Status1
  Header : Blocks_lib/Header  width=Landscape  addtext=''
  raptor_can_rxmsg : Raptor_lib/CAN/raptor_can_rxmsg  canDefinition=struct('dbcFile', 'BMS dbc file_rev4.0.dbc','message', 'HVES1_Status1','comment', '100ms','signals', {{'POS_Contact_State','PSV_ISO_TEST_State','HVIL_Status','HV_BUS_CONNECT_Status','OPERATIONAL_State'}},'enabled', [ 1 1 1 1 1;],'scaled', [ 1 1 1 1 1;],'canBus', 'bus','messageID', [ 217093875;],'idMask', [ 536870911;],'payloadMask', [],'payloadValue', [],'period', [ 0;],'mailbox', '''''','queueSize', [ 1;],'label', [ 1;],'ver', [ 2;],'showID', [ 0;],'showRaw', [ 0;],'showRawMsg', [ 0;],'showAge', [ 1;],'fill', [ 0;],'editID', [ 0;],'signalOrder', [ 3;],'signalAscDes', [ 1;])  canBus=bus  mailbox=''  payloadMask=[]  payloadValue=[]  idMask=hex2dec('1FFFFFFF')  queueSize=1  showID=0  label=1  fill=0  id=217093875  showRaw=0  showAge=1  signalOrder=3  signalInfo={{struct('Name', 'POS_Contact_State','Startbit', [ 0;],'SignalSize', [ 2;],'ByteOrder', 'LittleEndian','ValueType', 'UNSIGNED','Class', 'uint8','Signed', [ 0;],'Factor', [ 1;],'Offset', [ 0;],'Min', [ 0;],'Max', [ 3;],'Units', '','Comment', '','StartBit', [ 0;]),struct('Name', 'PSV_ISO_TEST_State','Startbit', [ 0;],'SignalSize', [ 4;],'ByteOrder', 'LittleEndian','ValueType', 'UNSIGNED','Class', 'uint8','Signed', [ 0;],'Factor', [ 1;],'Offset', [ 0;],'Min', [ 0;],'Max', [ 15;],'Units', '','Comment', '','StartBit', [ 16;]),struct('Name', 'HVIL_Status','Startbit', [ 0;],'SignalSize', [ 2;],'ByteOrder', 'LittleEndian','ValueType', 'UNSIGNED','Class', 'uint8','Signed', [ 0;],'Factor', [ 1;],'Offset', [ 0;],'Min', [ 0;],'Max', [ 3;],'Units', '','Comment', '','StartBit', [ 20;]),struct('Name', 'HV_BUS_CONNECT_Status','Startbit', [ 0;],'SignalSize', [ 4;],'ByteOrder', 'LittleEndian','ValueType', 'UNSIGNED','Class', 'uint8','Signed', [ 0;],'Factor', [ 1;],'Offset', [ 0;],'Min', [ 0;],'Max', [ 15;],'Units', '','Comment', '','StartBit', [ 40;]),struct('Name', 'OPERATIONAL_State','Startbit', [ 0;],'SignalSize', [ 4;],'ByteOrder', 'LittleEndian','ValueType', 'UNSIGNED','Class', 'uint8','Signed', [ 0;],'Factor', [ 1;],'Offset', [ 0;],'Min', [ 0;],'Max', [ 15;],'Units', '','Comment', '','StartBit', [ 44;])}}
      settings: SourceProductName=Raptor
  Data : Outport  VectorParamsAs1DForOutWhenUnconnected=off
  wires:
  Bus Creator/1 -> Data/1  "MsgName"
  raptor_can_rxmsg/2 -> CANRxField/1  "POS_Contact_State"
  CANRxMsgStatus/1 -> Bus Creator/1
  CANRxField/1 -> Bus Creator/2
  DiagEnbl/1 -> CANRxMsgStatus/1
  raptor_can_rxmsg/1 -> CANRxMsgStatus/2  "Age"
  raptor_can_rxmsg/3 -> CANRxField1/1  "PSV_ISO_TEST_State"
  raptor_can_rxmsg/4 -> CANRxField2/1  "HVIL_Status"
  CANRxField1/1 -> Bus Creator/3
  CANRxField2/1 -> Bus Creator/4
  raptor_can_rxmsg/5 -> CANRxField3/1  "HV_BUS_CONNECT_Status"
  raptor_can_rxmsg/6 -> CANRxField4/1  "OPERATIONAL_State"
  CANRxField3/1 -> Bus Creator/5
  CANRxField4/1 -> Bus Creator/6

== system VCMGCM1962020b_v2/Fgnd/Sensors/CAN/Battery/HVES_Current_Data ==
  DiagEnbl : Inport
  Bus Creator : BusCreator  Inputs=4
  CANRxField1 : Blocks_lib/CANRxField  typ='double'  custom=off  custom_nam='---'  custom_units='---'
  CANRxField2 : Blocks_lib/CANRxField  typ='double'  custom=off  custom_nam='---'  custom_units='---'
  CANRxField5 : Blocks_lib/CANRxField  typ='double'  custom=off  custom_nam='---'  custom_units='---'
  CANRxMsgStatus : Blocks_lib/CANRxMsgStatus  samptime=samptime  custom=off  custom_nam='Name'  msgnam=HVES_Current_Data
  Header : Blocks_lib/Header  width=Landscape  addtext=''
  raptor_can_rxmsg : Raptor_lib/CAN/raptor_can_rxmsg  canDefinition=struct('dbcFile', 'BMS dbc file_rev4.0.dbc','message', 'HVES_Current_Data','comment', '20ms','signals', {{'Batt_Curr','Batt_Chg_Curr_Lmt','Batt_Dchg_Curr_Lmt'}},'enabled', [ 1 1 1;],'scaled', [ 1 1 1;],'canBus', 'bus','messageID', [ 218042355;],'idMask', [ 536870911;],'payloadMask', [],'payloadValue', [],'period', [ 0;],'mailbox', '''''','queueSize', [ 1;],'label', [ 1;],'ver', [ 2;],'showID', [ 0;],'showRaw', [ 0;],'showRawMsg', [ 0;],'showAge', [ 1;],'fill', [ 0;],'editID', [ 0;],'signalOrder', [ 3;],'signalAscDes', [ 1;])  canBus=bus  mailbox=''  payloadMask=[]  payloadValue=[]  idMask=hex2dec('1FFFFFFF')  queueSize=1  showID=0  label=1  fill=0  id=218042355  showRaw=0  showAge=1  signalOrder=3  signalInfo={{struct('Name', 'Batt_Curr','Startbit', [ 0;],'SignalSize', [ 16;],'ByteOrder', 'LittleEndian','ValueType', 'UNSIGNED','Class', 'uint16','Signed', [ 0;],'Factor', [ 0.1;],'Offset', [ 3212.7;],'Min', [ -3212.7;],'Max', [ 3212.7;],'Units', 'A','Comment', '','StartBit', [ 0;]),struct('Name', 'Batt_Chg_Curr_Lmt','Startbit', [ 0;],'SignalSize', [ 16;],'ByteOrder', 'LittleEndian','ValueType', 'UNSIGNED','Class', 'uint16','Signed', [ 0;],'Factor', [ 0.1;],'Offset', [ 3212.7;],'Min', [ -3212.7;],'Max', [ 3212.7;],'Units', 'A','Comment', '','StartBit', [ 16;]),struct('Name', 'Batt_Dchg_Curr_Lmt','Startbit', [ 0;],'SignalSize', [ 16;],'ByteOrder', 'LittleEndian','ValueType', 'UNSIGNED','Class', 'uint16','Signed', [ 0;],'Factor', [ 0.1;],'Offset', [ 3212.7;],'Min', [ -3212.7;],'Max', [ 3212.7;],'Units', 'A','Comment', '','StartBit', [ 32;])}}
      settings: SourceProductName=Raptor
  Data : Outport  VectorParamsAs1DForOutWhenUnconnected=off
  wires:
  Bus Creator/1 -> Data/1  "MsgName"
  CANRxMsgStatus/1 -> Bus Creator/1
  DiagEnbl/1 -> CANRxMsgStatus/1
  raptor_can_rxmsg/1 -> CANRxMsgStatus/2  "Age"
  raptor_can_rxmsg/2 -> CANRxField5/1  "Batt_Curr"
  raptor_can_rxmsg/3 -> CANRxField1/1  "Batt_Chg_Curr_Lmt"
  raptor_can_rxmsg/4 -> CANRxField2/1  "Batt_Dchg_Curr_Lmt"
  CANRxField5/1 -> Bus Creator/2
  CANRxField1/1 -> Bus Creator/3
  CANRxField2/1 -> Bus Creator/4

== system VCMGCM1962020b_v2/Fgnd/Sensors/CAN/Battery/HVES_Op_State ==
  DiagEnbl : Inport
  Bus Creator : BusCreator  Inputs=4
  CANRxField : Blocks_lib/CANRxField  typ='uint8'  custom=off  custom_nam='---'  custom_units='---'
  CANRxField1 : Blocks_lib/CANRxField  typ='uint8'  custom=off  custom_nam='---'  custom_units='---'
  CANRxField2 : Blocks_lib/CANRxField  typ='uint8'  custom=off  custom_nam='---'  custom_units='---'
  CANRxMsgStatus : Blocks_lib/CANRxMsgStatus  samptime=samptime  custom=off  custom_nam='Name'  msgnam=HVES_Op_State
  Header : Blocks_lib/Header  width=Landscape  addtext=''
  raptor_can_rxmsg : Raptor_lib/CAN/raptor_can_rxmsg  canDefinition=struct('dbcFile', 'BMS dbc file_rev4.0.dbc','message', 'HVES_Op_State','comment', '100ms','signals', {{'Prev_Op_State','Curr_Op_State','Next_Op_State'}},'enabled', [ 1 1 1;],'scaled', [ 1 1 1;],'canBus', 'bus','messageID', [ 218038771;],'idMask', [ 536870911;],'payloadMask', [],'payloadValue', [],'period', [ 0;],'mailbox', '''''','queueSize', [ 1;],'label', [ 1;],'ver', [ 2;],'showID', [ 0;],'showRaw', [ 0;],'showRawMsg', [ 0;],'showAge', [ 1;],'fill', [ 0;],'editID', [ 0;],'signalOrder', [ 3;],'signalAscDes', [ 1;])  canBus=bus  mailbox=''  payloadMask=[]  payloadValue=[]  idMask=hex2dec('1FFFFFFF')  queueSize=1  showID=0  label=1  fill=0  id=218038771  showRaw=0  showAge=1  signalOrder=3  signalInfo={{struct('Name', 'Prev_Op_State','Startbit', [ 0;],'SignalSize', [ 4;],'ByteOrder', 'LittleEndian','ValueType', 'UNSIGNED','Class', 'uint8','Signed', [ 0;],'Factor', [ 1;],'Offset', [ 0;],'Min', [ 0;],'Max', [ 15;],'Units', '','Comment', '','StartBit', [ 0;]),struct('Name', 'Curr_Op_State','Startbit', [ 0;],'SignalSize', [ 4;],'ByteOrder', 'LittleEndian','ValueType', 'UNSIGNED','Class', 'uint8','Signed', [ 0;],'Factor', [ 1;],'Offset', [ 0;],'Min', [ 0;],'Max', [ 15;],'Units', '','Comment', '','StartBit', [ 4;]),struct('Name', 'Next_Op_State','Startbit', [ 0;],'SignalSize', [ 4;],'ByteOrder', 'LittleEndian','ValueType', 'UNSIGNED','Class', 'uint8','Signed', [ 0;],'Factor', [ 1;],'Offset', [ 0;],'Min', [ 0;],'Max', [ 15;],'Units', '','Comment', '','StartBit', [ 8;])}}
      settings: SourceProductName=Raptor
  Data : Outport  VectorParamsAs1DForOutWhenUnconnected=off
  wires:
  Bus Creator/1 -> Data/1  "MsgName"
  raptor_can_rxmsg/2 -> CANRxField/1  "Prev_Op_State"
  CANRxMsgStatus/1 -> Bus Creator/1
  CANRxField/1 -> Bus Creator/2
  DiagEnbl/1 -> CANRxMsgStatus/1
  raptor_can_rxmsg/1 -> CANRxMsgStatus/2  "Age"
  raptor_can_rxmsg/3 -> CANRxField1/1  "Curr_Op_State"
  raptor_can_rxmsg/4 -> CANRxField2/1  "Next_Op_State"
  CANRxField1/1 -> Bus Creator/3
  CANRxField2/1 -> Bus Creator/4

== system VCMGCM1962020b_v2/Fgnd/Sensors/CAN/Battery/HVES_Stress ==
  DiagEnbl : Inport
  Bus Creator : BusCreator  Inputs=5
  CANRxField{1..3,5} (4 alike) : Blocks_lib/CANRxField  typ='double'  custom=off  custom_nam='---'  custom_units='---'
  CANRxMsgStatus : Blocks_lib/CANRxMsgStatus  samptime=samptime  custom=off  custom_nam='Name'  msgnam=HVES_Stress
  Header : Blocks_lib/Header  width=Landscape  addtext=''
  raptor_can_rxmsg : Raptor_lib/CAN/raptor_can_rxmsg  canDefinition=struct('dbcFile', 'BMS dbc file_rev4.0.dbc','message', 'HVES_Stress','comment', '100ms','signals', {{'Chg_Stress_Estimate','Dchg_Stress_Estimate','Allowed_Charge_Time','Allowed_Discharge_Time'}},'enabled', [ 1 1 1 1;],'scaled', [ 1 1 1 1;],'canBus', 'bus','messageID', [ 218039027;],'idMask', [ 536870911;],'payloadMask', [],'payloadValue', [],'period', [ 0;],'mailbox', '''''','queueSize', [ 1;],'label', [ 1;],'ver', [ 2;],'showID', [ 0;],'showRaw', [ 0;],'showRawMsg', [ 0;],'showAge', [ 1;],'fill', [ 0;],'editID', [ 0;],'signalOrder', [ 3;],'signalAscDes', [ 1;])  canBus=bus  mailbox=''  payloadMask=[]  payloadValue=[]  idMask=hex2dec('1FFFFFFF')  queueSize=1  showID=0  label=1  fill=0  id=218039027  showRaw=0  showAge=1  signalOrder=3  signalInfo={{struct('Name', 'Chg_Stress_Estimate','Startbit', [ 0;],'SignalSize', [ 16;],'ByteOrder', 'LittleEndian','ValueType', 'UNSIGNED','Class', 'uint16','Signed', [ 0;],'Factor', [ 0.001;],'Offset', [ 0;],'Min', [ 0;],'Max', [ 1;],'Units', '','Comment', '','StartBit', [ 0;]),struct('Name', 'Dchg_Stress_Estimate','Startbit', [ 0;],'SignalSize', [ 16;],'ByteOrder', 'LittleEndian','ValueType', 'UNSIGNED','Class', 'uint16','Signed', [ 0;],'Factor', [ 0.001;],'Offset', [ 0;],'Min', [ 0;],'Max', [ 1;],'Units', '','Comment', '','StartBit', [ 16;]),struct('Name', 'Allowed_Charge_Time','Startbit', [ 0;],'SignalSize', [ 16;],'ByteOrder', 'LittleEndian','ValueType', 'UNSIGNED','Class', 'uint16','Signed', [ 0;],'Factor', [ 0.1;],'Offset', [ -2;],'Min', [ 0;],'Max', [ 0;],'Units', 's','Comment', '','StartBit', [ 32;]),struct('Name', 'Allowed_Discharge_Time','Startbit', [ 0;],'SignalSize', [ 16;],'ByteOrder', 'LittleEndian','ValueType', 'UNSIGNED','Class', 'uint16','Signed', [ 0;],'Factor', [ 0.1;],'Offset', [ -2;],'Min', [ 0;],'Max', [ 0;],'Units', 's','Comment', '','StartBit', [ 48;])}}
      settings: SourceProductName=Raptor
  Data : Outport  VectorParamsAs1DForOutWhenUnconnected=off
  wires:
  Bus Creator/1 -> Data/1  "MsgName"
  CANRxMsgStatus/1 -> Bus Creator/1
  DiagEnbl/1 -> CANRxMsgStatus/1
  raptor_can_rxmsg/1 -> CANRxMsgStatus/2  "Age"
  raptor_can_rxmsg/2 -> CANRxField5/1  "Chg_Stress_Estimate"
  raptor_can_rxmsg/3 -> CANRxField1/1  "Dchg_Stress_Estimate"
  raptor_can_rxmsg/4 -> CANRxField2/1  "Allowed_Charge_Time"
  CANRxField5/1 -> Bus Creator/2
  CANRxField1/1 -> Bus Creator/3
  CANRxField2/1 -> Bus Creator/4
  raptor_can_rxmsg/5 -> CANRxField3/1  "Allowed_Discharge_Time"
  CANRxField3/1 -> Bus Creator/5

== system VCMGCM1962020b_v2/Fgnd/Sensors/CAN/Battery/HVES_Warranty ==
  DiagEnbl : Inport
  Bus Creator : BusCreator  Inputs=2
  CANRxField5 : Blocks_lib/CANRxField  typ='double'  custom=off  custom_nam='---'  custom_units='---'
  CANRxMsgStatus : Blocks_lib/CANRxMsgStatus  samptime=samptime  custom=off  custom_nam='Name'  msgnam=HVES_Warranty
  Header : Blocks_lib/Header  width=Landscape  addtext=''
  raptor_can_rxmsg : Raptor_lib/CAN/raptor_can_rxmsg  canDefinition=struct('dbcFile', 'BMS dbc file_rev4.0.dbc','message', 'HVES_Warranty','comment', '100ms','signals', {{'Warranty_Remaining'}},'enabled', [ 1;],'scaled', [ 1;],'canBus', 'bus','messageID', [ 218038515;],'idMask', [ 536870911;],'payloadMask', [],'payloadValue', [],'period', [ 0;],'mailbox', '''''','queueSize', [ 1;],'label', [ 1;],'ver', [ 2;],'showID', [ 0;],'showRaw', [ 0;],'showRawMsg', [ 0;],'showAge', [ 1;],'fill', [ 0;],'editID', [ 0;],'signalOrder', [ 3;],'signalAscDes', [ 1;])  canBus=bus  mailbox=''  payloadMask=[]  payloadValue=[]  idMask=hex2dec('1FFFFFFF')  queueSize=1  showID=0  label=1  fill=0  id=218038515  showRaw=0  showAge=1  signalOrder=3  signalInfo={{struct('Name', 'Warranty_Remaining','Startbit', [ 0;],'SignalSize', [ 32;],'ByteOrder', 'LittleEndian','ValueType', 'UNSIGNED','Class', 'uint32','Signed', [ 0;],'Factor', [ 1;],'Offset', [ 0;],'Min', [ 0;],'Max', [ 0;],'Units', 'Ah','Comment', '','StartBit', [ 32;])}}
      settings: SourceProductName=Raptor
  Data : Outport  VectorParamsAs1DForOutWhenUnconnected=off
  wires:
  Bus Creator/1 -> Data/1  "MsgName"
  CANRxMsgStatus/1 -> Bus Creator/1
  DiagEnbl/1 -> CANRxMsgStatus/1
  raptor_can_rxmsg/1 -> CANRxMsgStatus/2  "Age"
  raptor_can_rxmsg/2 -> CANRxField5/1  "Warranty_Remaining"
  CANRxField5/1 -> Bus Creator/2

== system VCMGCM1962020b_v2/Fgnd/Sensors/CAN/Battery/MsgName ==
  DiagEnbl : Inport
  Bus Creator : BusCreator  Inputs=2
  CANRxField : Blocks_lib/CANRxField  typ='boolean'  custom=off  custom_nam='---'  custom_units='---'
  CANRxMsgStatus : Blocks_lib/CANRxMsgStatus  samptime=samptime  custom=off  custom_nam='Name'  msgnam=Batt_Module_Volt_Delta
  Header : Blocks_lib/Header  width=Landscape  addtext=''
  raptor_can_rxmsg : Raptor_lib/CAN/raptor_can_rxmsg  canDefinition=struct('dbcFile', 'BMS dbc file_rev6.0.dbc','message', 'Batt_Module_Volt_Delta','comment', '','signals', {{'Voltage_Delta_Mod_0'}},'enabled', [ 1;],'scaled', [ 1;],'canBus', 'bus','messageID', [ 218039283;],'idMask', [ 536870911;],'payloadMask', [],'payloadValue', [],'period', [ 0;],'mailbox', '''''','queueSize', [ 1;],'label', [ 1;],'ver', [ 2;],'showID', [ 0;],'showRaw', [ 0;],'fill', [ 0;],'editID', [ 0;],'signalOrder', [ 3;],'signalAscDes', [ 1;])  canBus=bus  mailbox=''  payloadMask=[]  payloadValue=[]  idMask=hex2dec('1FFFFFFF')  queueSize=1  showID=0  label=1  fill=0  id=218039283  showRaw=0  showAge=1  signalOrder=3  signalInfo={{struct('Name', 'Voltage_Delta_Mod_0','Startbit', [ 0;],'SignalSize', [ 16;],'ByteOrder', 'LittleEndian','ValueType', 'UNSIGNED','Class', 'uint16','Signed', [ 0;],'Factor', [ 0.1;],'Offset', [ 0;],'Min', [ 0;],'Max', [ 6553.6;],'Units', 'V','Comment', '','StartBit', [ 0;])}}
      settings: SourceProductName=Raptor
  Data : Outport  VectorParamsAs1DForOutWhenUnconnected=off
  wires:
  Bus Creator/1 -> Data/1  "MsgName"
  raptor_can_rxmsg/2 -> CANRxField/1  "Voltage_Delta_Mod_0"
  CANRxMsgStatus/1 -> Bus Creator/1
  CANRxField/1 -> Bus Creator/2
  DiagEnbl/1 -> CANRxMsgStatus/1
  raptor_can_rxmsg/1 -> CANRxMsgStatus/2  "Age"
